simulink model "EvPowertrainController2EM"  (R2023a)
settings: configuration reference "VehicleFixed10ms" (kept outside this file)
model workspace (MAT data in the model file):
  CtrlVcuCnstrntPnltyFctr = 10000000
  CtrlVcuEMTrqSplitGrid = 200
  CtrlVcuPwrDeltaPnlty = 2
  CtrlVcuTracPwrErrPnlty = 6
  CtrlVcuTrqVecBrkThresh = 0.01
  CtrlVcuTrqVecIGain = 0
  CtrlVcuTrqVecMinTrq = 50
  CtrlVcuTrqVecPGain = -2000
  CtrlVcuTrqVecSteerThresh = 0.349065850399
  CtrlVcuTrqVecVelThresh = 2.5
undefined symbols (not defined in the file): CtrlVcuEvChrgLmtBpt, CtrlVcuEvRegenBrkCutOff, CtrlVcuEvSocBpt, eff, PlntBrkActrBoreFrnt, PlntBrkFrntBias, PlntBrkKinFricCffFrnt, PlntBrkNumPadsFrnt, PlntBrkPadMeanRadiusFrnt, PlntBrkPrsFctr, PlntBrkRearBias, PlntDiffrntl2Eff, PlntDiffrntl2Ratio, PlntDiffrntlEff, PlntDiffrntlRatio, PlntEM1EffTbl, PlntEM1Spd, PlntEM1Trq, PlntEM1TrqEff, PlntEM2EffTbl, PlntEM2Spd, PlntEM2Trq, PlntEM2TrqEff, PlntEM3EffTbl, PlntEM3Spd, PlntEM3Trq, PlntEM3TrqEff, PlntEMWhlGearEffFL, PlntEMWhlGearEffRL, PlntEMWhlGearRatioFL, PlntEMWhlGearRatioRL, PlntTransEffSpdBpt, PlntTransEffTbl, PlntTransEffTempBpt, PlntTransEffTrqBpt, PlntTransGearNumVect, PlntTransGearRatioVect, PlntVehDstCGFrntAxl, PlntVehDstCGRearAxl, PlntWhlLdRadius, RegenEnd, RegenStrt
libraries: simulink x13, autolibutils x2, slpidlib x2
(part 5 of 5)

== system EvPowertrainController2EM/Energy Management/Powertrain Constraints /EM Constraint Rear/Tabular Power Loss Data/2EM/WhlTrq2EMTrq/Diff Eta ==
  note: Pwr >= 0, v = 1
      | Pwr < 0, v= -1
  SpdIn : Inport
  TrqIn : Inport  Port=2
  Constant : Constant  Value=PlntDiffrntl2Eff
  Constant1 : Constant  SampleTime=-1
  Constant2 : Constant  Value=-1  SampleTime=-1
  Math Function1 : Math  Operator=pow  SignedPower=on  OutputSignalType=real
  Product1 : Product
  Switch2 : Switch  SaturateOnIntegerOverflow=off  InputSameDT=off
  eta : Outport  VectorParamsAs1DForOutWhenUnconnected=off
  wires:
  SpdIn/1 -> Product1/2
  Constant/1 -> Math Function1/1
  Constant2/1 -> Switch2/3
  Constant1/1 -> Switch2/1
  Product1/1 -> Switch2/2
  Switch2/1 -> Math Function1/2
  Math Function1/1 -> eta/1
  TrqIn/1 -> Product1/1

== system EvPowertrainController2EM/Energy Management/Powertrain Constraints /EM Constraint Rear/Tabular Power Loss Data/3EM Dual Front/WhlTrq2EMTrq/Diff Eta ==
  note: Pwr >= 0, v = 1
      | Pwr < 0, v= -1
  SpdIn : Inport
  TrqIn : Inport  Port=2
  Constant : Constant  Value=PlntDiffrntl2Eff
  Constant1 : Constant  SampleTime=-1
  Constant2 : Constant  Value=-1  SampleTime=-1
  Math Function1 : Math  Operator=pow  SignedPower=on  OutputSignalType=real
  Product1 : Product
  Switch2 : Switch  SaturateOnIntegerOverflow=off  InputSameDT=off
  eta : Outport  VectorParamsAs1DForOutWhenUnconnected=off
  wires:
  TrqIn/1 -> Product1/1
  Math Function1/1 -> eta/1
  Switch2/1 -> Math Function1/2
  Product1/1 -> Switch2/2
  Constant1/1 -> Switch2/1
  Constant2/1 -> Switch2/3
  Constant/1 -> Math Function1/1
  SpdIn/1 -> Product1/2

== system EvPowertrainController2EM/Energy Management/Powertrain Constraints /EM Constraint Rear/Tabular Power Loss Data/3EM Dual Rear or 4EM/WhlTrq2EMTrq/Gear Eta ==
  note: Pwr >= 0, v = 1
      | Pwr < 0, v= -1
  SpdIn : Inport
  TrqIn : Inport  Port=2
  Constant : Constant  Value=PlntEMWhlGearEffRL
  Constant1 : Constant  SampleTime=-1
  Constant2 : Constant  Value=-1  SampleTime=-1
  Math Function1 : Math  Operator=pow  SignedPower=on  OutputSignalType=real
  Product1 : Product
  Switch2 : Switch  SaturateOnIntegerOverflow=off  InputSameDT=off
  eta : Outport  VectorParamsAs1DForOutWhenUnconnected=off
  wires:
  TrqIn/1 -> Product1/1
  Math Function1/1 -> eta/1
  Switch2/1 -> Math Function1/2
  Product1/1 -> Switch2/2
  Constant1/1 -> Switch2/1
  Constant2/1 -> Switch2/3
  Constant/1 -> Math Function1/1
  SpdIn/1 -> Product1/2

== matlab function EvPowertrainController2EM/Energy Management/Hamiltonian computation and minimization/MATLAB Function ==
  data: minH output; idx output; H input; InfFlag input; allInf output
function [minH, idx, allInf] = fcn(H, InfFlag)

if all(InfFlag) 
    [minH, idx] = min(H);
    allInf = 1;
else
    [minH, idx] = min(H);
    allInf = 0;
end

== matlab function EvPowertrainController2EM/Torque Vectoring/4EM/Torque Vectoring Split Function Front ==
  data: MaxTrq input; TrqLeftOut output; TrqLeft input; TrqRght input; TrqRghtOut output; TrqVec input; Enbl input; BrkThresh input; MinTrq input
function [TrqLeftOut, TrqRghtOut] = fcn(MaxTrq, TrqLeft, TrqRght, TrqVec, Enbl, BrkThresh, MinTrq)
% Enbl:= flag to turn on TV, true if steering wheel is turned and non-zero vehicle speed
% BrkThresh:= flag to turn on TV, true if not braking
TrqLmt = min(MaxTrq-abs(TrqLeft),MaxTrq-abs(TrqRght));
DeltaTrq = min(MinTrq, min(TrqLmt,abs(TrqVec)))*sign(TrqVec)*Enbl;% limit difference in torque between tires to +/-MinTrq and to max/min motor torque
if BrkThresh > 0 % Not braking. Use Torque vectoring
    TrqLeftOut = (TrqLeft+DeltaTrq);
    TrqRghtOut = (TrqRght-DeltaTrq);
else % ignore TV
    TrqLeftOut = TrqLeft;
    TrqRghtOut = TrqRght;
end

== matlab function EvPowertrainController2EM/Torque Vectoring/3EM/Torque Vectoring Split Function ==
  data: MaxTrq input; TrqLeftOut output; TrqLeft input; TrqRght input; TrqRghtOut output; TrqVec input; Enbl input; BrkThresh input; MinTrq input
function [TrqLeftOut, TrqRghtOut] = fcn(MaxTrq, TrqLeft, TrqRght, TrqVec, Enbl, BrkThresh, MinTrq)
% Enbl:= flag to turn on TV, true if steering wheel is turned and non-zero vehicle speed
% BrkThresh:= flag to turn on TV, true if not braking
TrqLmt = min(MaxTrq-abs(TrqLeft),MaxTrq-abs(TrqRght));
DeltaTrq = min(MinTrq, min(TrqLmt,abs(TrqVec)))*sign(TrqVec)*Enbl;% limit difference in torque between tires to +/-MinTrq and to max/min motor torque
if BrkThresh > 0 % Not braking. Use Torque vectoring
    TrqLeftOut = (TrqLeft+DeltaTrq);
    TrqRghtOut = (TrqRght-DeltaTrq);
else % ignore TV
    TrqLeftOut = TrqLeft;
    TrqRghtOut = TrqRght;
end

== matlab function EvPowertrainController2EM/Torque Vectoring/4EM/Torque Vectoring Split Function Rear ==
  data: MaxTrq input; TrqLeftOut output; TrqLeft input; TrqRght input; TrqRghtOut output; TrqVec input; Enbl input; BrkThresh input; MinTrq input
function [TrqLeftOut, TrqRghtOut] = fcn(MaxTrq, TrqLeft, TrqRght, TrqVec, Enbl, BrkThresh, MinTrq)
% Enbl:= flag to turn on TV, true if steering wheel is turned and non-zero vehicle speed
% BrkThresh:= flag to turn on TV, true if not braking
TrqLmt = min(MaxTrq-abs(TrqLeft),MaxTrq-abs(TrqRght));
DeltaTrq = min(MinTrq, min(TrqLmt,abs(TrqVec)))*sign(TrqVec)*Enbl;% limit difference in torque between tires to +/-MinTrq and to max/min motor torque
if BrkThresh > 0 % Not braking. Use Torque vectoring
    TrqLeftOut = (TrqLeft+DeltaTrq);
    TrqRghtOut = (TrqRght-DeltaTrq);
else % ignore TV
    TrqLeftOut = TrqLeft;
    TrqRghtOut = TrqRght;
end
